simulink model "simulacaoProcesso1"  (Simulink 9.1)
settings: Solver=VariableStepAuto  StartTime=0.0  StopTime=10.0  RelTol=1e-3  EnableMultiTasking=on
settings Model: SuppressorTable=22 serialization::archive 11 0 6 0 0 0 1 0  Creator=thiag  LastModifiedBy=gshimabuko
settings SolverCC: ZeroCrossAlgorithm=Adaptive
settings DataIOCC: SaveFormat=Dataset
settings DebuggingCC: UnderspecifiedInitializationDetection=Simplified  MergeDetectMultiDrivingBlocksExec=error  MaxConsecutiveZCsMsg=none
settings HardwareCC: ProdBitPerPointer=64  ProdBitPerSizeT=64  ProdBitPerPtrDiffT=64  ProdLargestAtomicFloat=Float  ProdIntDivRoundTo=Zero  ProdEndianess=LittleEndian  ProdWordSize=64  ProdHWDeviceType=Intel->x86-64 (Windows64)
settings ModelReferenceCC: PropagateSignalLabelsOutOfModel=on
settings GRTTargetCC: GeneratePreprocessorConditionals=Disable all  CombineOutputUpdateFcns=on  GRTInterface=off

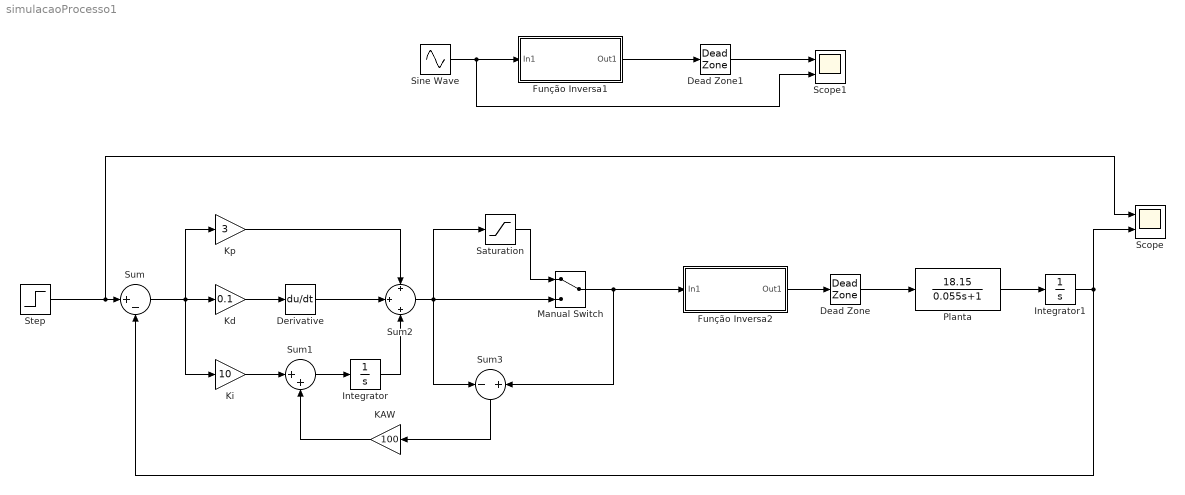
== system simulacaoProcesso1 ==
  Dead Zone : DeadZone  LowerValue=-0.7  UpperValue=0.95  SaturateOnIntegerOverflow=on
  Dead Zone1 : DeadZone  LowerValue=-0.7  UpperValue=0.95  SaturateOnIntegerOverflow=on
  Derivative : Derivative
  Função Inversa1 : Subsystem
  Função Inversa2 : Subsystem
  Integrator : Integrator
  Integrator1 : Integrator
  KAW : Gain  Gain=100
  Kd : Gain  Gain=0.1
  Ki : Gain  Gain=10
  Kp : Gain  Gain=3
  Manual Switch : ManualSwitch
  Planta : TransferFcn  Numerator=[18.15]  Denominator=[0.055 1]
  Saturation : Saturate  UpperLimit=7.2  LowerLimit=-7.2
  Scope : Scope  NumInputPorts=2
  Scope1 : Scope  NumInputPorts=2
  Sine Wave : Sin  Amplitude=5  Frequency=6.28  SampleTime=0
  Step : Step  After=5  SampleTime=0
  Sum : Sum  Inputs=|+-
  Sum1 : Sum  Inputs=|++
  Sum2 : Sum  Inputs=+|+|+
  Sum3 : Sum  Inputs=-+
  wires:
  Kd/1 -> Derivative/1
  Ki/1 -> Sum1/1
  Sum1/1 -> Integrator/1
  Integrator/1 -> Sum2/3
  Derivative/1 -> Sum2/2
  Kp/1 -> Sum2/1
  Manual Switch/1 -> Sum3/2, Função Inversa2/1(In1)
  Sum/1 -> Ki/1, Kp/1, Kd/1
  Planta/1 -> Integrator1/1
  Integrator1/1 -> Sum/2, Scope/2
  Step/1 -> Scope/1, Sum/1
  Função Inversa2/1(Out1) -> Dead Zone/1
  Função Inversa1/1(Out1) -> Dead Zone1/1
  Dead Zone1/1 -> Scope1/1
  Sine Wave/1 -> Scope1/2, Função Inversa1/1(In1)
  Saturation/1 -> Manual Switch/1
  Sum2/1 -> Sum3/1, Manual Switch/2, Saturation/1
  Sum3/1 -> KAW/1
  KAW/1 -> Sum1/2
  Dead Zone/1 -> Planta/1

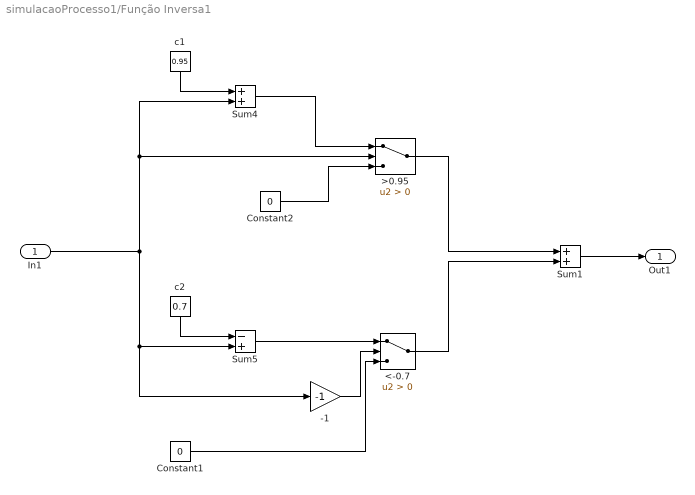
== system simulacaoProcesso1/Função Inversa1 ==
  In1 : Inport
  -1 : Gain  Gain=-1
  "<-0.7 " : Switch  Criteria=u2 > Threshold
  ">0.95 " : Switch  Criteria=u2 > Threshold
  Constant1 : Constant  Value=0
  Constant2 : Constant  Value=0
  Sum1 : Sum
  Sum4 : Sum
  Sum5 : Sum  Inputs=-+
  c1 : Constant  Value=0.95
  c2 : Constant  Value=0.7
  Out1 : Outport
  wires:
  c2/1 -> Sum5/1
  In1/1 -> Sum4/2, ">0.95 "/2, -1/1, Sum5/2
  -1/1 -> "<-0.7 "/2
  Sum5/1 -> "<-0.7 "/1
  Constant1/1 -> "<-0.7 "/3
  "<-0.7 "/1 -> Sum1/2
  ">0.95 "/1 -> Sum1/1
  Sum1/1 -> Out1/1
  c1/1 -> Sum4/1
  Sum4/1 -> ">0.95 "/1
  Constant2/1 -> ">0.95 "/3

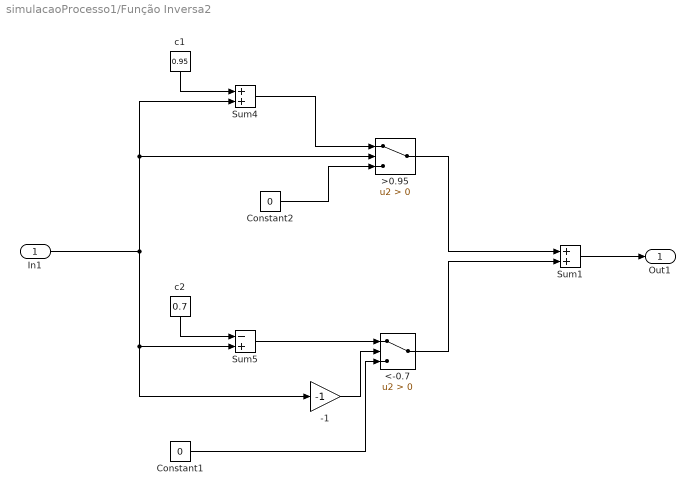
== system simulacaoProcesso1/Função Inversa2 ==
  In1 : Inport
  -1 : Gain  Gain=-1
  "<-0.7 " : Switch  Criteria=u2 > Threshold
  ">0.95 " : Switch  Criteria=u2 > Threshold
  Constant1 : Constant  Value=0
  Constant2 : Constant  Value=0
  Sum1 : Sum
  Sum4 : Sum
  Sum5 : Sum  Inputs=-+
  c1 : Constant  Value=0.95
  c2 : Constant  Value=0.7
  Out1 : Outport
  wires:
  c2/1 -> Sum5/1
  In1/1 -> Sum4/2, ">0.95 "/2, -1/1, Sum5/2
  -1/1 -> "<-0.7 "/2
  Sum5/1 -> "<-0.7 "/1
  Constant1/1 -> "<-0.7 "/3
  "<-0.7 "/1 -> Sum1/2
  ">0.95 "/1 -> Sum1/1
  Sum1/1 -> Out1/1
  c1/1 -> Sum4/1
  Sum4/1 -> ">0.95 "/1
  Constant2/1 -> ">0.95 "/3
